simulink model "complete_plant"  (R2021b)
settings: Solver=VariableStepAuto  StartTime=0.0  StopTime=15  RelTol=1e-3
values from neighbouring files (symbols this model uses):
  a = Simulink.Parameter(1.14)    [startup.m]
  A1 = Simulink.Parameter(39.8344)    [startup.m]
  A2 = Simulink.Parameter(813.0780)    [startup.m]
  b = Simulink.Parameter(-0.03291)    [startup.m]
  B1 = Simulink.Parameter(0.000001287)    [startup.m]
  B2 = Simulink.Parameter(-0.002325)    [startup.m]
  B3 = Simulink.Parameter(3.797)    [startup.m]
  c = Simulink.Parameter(-1.14)    [startup.m]
  C1 = Simulink.Parameter(-0.000000002541)    [startup.m]
  C2 = Simulink.Parameter(0.000005279)    [startup.m]
  C3 = Simulink.Parameter(-0.003943)    [startup.m]
  C4 = Simulink.Parameter(3.634)    [startup.m]
  C_param = Simulink.Parameter([0 13757.41 21278.97 26666.02 30253.47 30313.18 30313.18])    [startup.m]
  d = Simulink.Parameter(-1.027)    [startup.m]
  driver_gain = 1    [startup.m]
  FZ_C = Simulink.Parameter([0 204.13 427.04 668.1 895.72 1124.40 1324.40])    [startup.m]
  gr = Simulink.Parameter([6.63043, 6.63043, 7.95652, 7.95652])    [startup.m]
  I = 15    [startup.m]
  inch2mm = Simulink.Parameter(25.4)    [startup.m]
  J_z = Simulink.Parameter(75)    [startup.m]
  k_limit = Simulink.Parameter(3.461)    [startup.m]
  Ku = Simulink.Parameter(0.24 / g.Value)    [startup.m]
  l = Simulink.Parameter([0.7922471, 0.7828529])    [startup.m]
  max_yaw_field = Simulink.Parameter([1.34 1.34 1.34 1.66 1.14 1.24 0.754 0.849 0.85 0.85])    [startup.m]
  min_speed_regen = Simulink.Parameter(85)    [startup.m]
  motor_efficiency = Simulink.Parameter([0.85, 0.85, 0.85, 0.85])    [startup.m]
  motor_limit_power = Simulink.Parameter([15000, 15000, 15000, 15000])    [startup.m]
  motor_limit_torque = Simulink.Parameter([-25, 25])    [startup.m]
  mu_factor = Simulink.Parameter(2/3)    [startup.m]
  P = 1    [startup.m]
  ramp_rate = 1    [startup.m]
  RE = Simulink.Parameter(0.2228169203)    [startup.m]
  s = Simulink.Parameter([0.647895, 0.62102])    [startup.m]
  S1 = Simulink.Parameter(7 * (10^(-5)))    [startup.m]
  S2 = Simulink.Parameter(-0.0038)    [startup.m]
  S3 = Simulink.Parameter(0.6535)    [startup.m]
  S4 = Simulink.Parameter(0.1061)    [startup.m]
  steer_slope = Simulink.Parameter(0.0111)    [startup.m]
  T = 0    [startup.m]
  T2F = Simulink.Parameter(single([29 29 35 35]))    [startup.m]
  tau = Simulink.Parameter(0)    [startup.m]
  time_delay = 0.022    [startup.m]
  V_target = Simulink.Parameter([0 3 6 9 12 15 18 21 25 31])    [startup.m]
undefined symbols (not defined in the file or in its folder): DiscIntNeverNeededParam
libraries: fl_lib x20, nesl_utility x12, sdl_lib x4, slpidlib x2, simulink x2, autolibdatasheetbattery x1, autolibmappedmotor x1, vehdynlibtire x1, autolibshared x1, vehdynlibviscommon x1
(part 3 of 4)

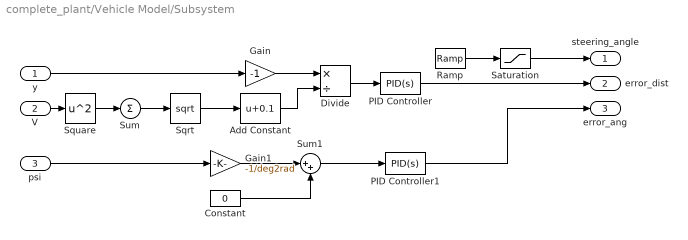
== system complete_plant/Vehicle Model/Subsystem ==
  y : Inport
  V : Inport  Port=2
  psi : Inport  Port=3
  Add Constant : Bias  Bias=0.1
  Constant : Constant  Value=0
  Divide : Product  Inputs=*/
  Gain : Gain  Gain=-1
  Gain1 : Gain  Gain=-1/deg2rad
  PID Controller : slpidlib/PID Controller  Controller=PID  Form=Parallel  TimeDomain=Continuous-time  UseExternalTs=off  SampleTime=-1  IntegratorMethod=Forward Euler  FilterMethod=Forward Euler  ControllerParametersSource=internal  P=50  I=0  D=2  UseFilter=on  N=50  TunerSelectOption=Transfer Function Based (PID Tuner App)  InitialConditionSource=internal  InitialConditionForIntegrator=0  InitialConditionForFilter=0  DifferentiatorICPrevScaledInput=0  ExternalReset=none  TrackingMode=off  Kt=1  LimitOutput=on  SatLimitsSource=internal  UpperSaturationLimit=40  LowerSaturationLimit=-40  LinearizeAsGain=on  AntiWindupMode=none  Kb=1  POutMin=[]  POutMax=[]  IOutMin=[]  IOutMax=[]  DOutMin=[]  DOutMax=[]  NOutMin=[]  NOutMax=[]  SumOutMin=[]  SumOutMax=[]  SaturationOutMin=[]  SaturationOutMax=[]  PParamMin=[]  PParamMax=[]  IParamMin=[]  IParamMax=[]  DParamMin=[]  DParamMax=[]  NParamMin=[]  NParamMax=[]  KbParamMin=[]  KbParamMax=[]  KtParamMin=[]  KtParamMax=[]  KbOutMin=[]  KbOutMax=[]  KtOutMin=[]  KtOutMax=[]  IntegratorOutMin=[]  IntegratorOutMax=[]  FilterOutMin=[]  FilterOutMax=[]  SumI1OutMin=[]  SumI1OutMax=[]  SumI2OutMin=[]  SumI2OutMax=[]  SumI3OutMin=[]  SumI3OutMax=[]  SumI4OutMin=[]  SumI4OutMax=[]  SumDOutMin=[]  SumDOutMax=[]  DifferentiatorOutMin=[]  DifferentiatorOutMax=[]  FilterDiffOutCoefMin=[]  FilterDiffOutCoefMax=[]  ReciprocalOutMin=[]  ReciprocalOutMax=[]  SumDenOutMin=[]  SumDenOutMax=[]  SumNumOutMin=[]  SumNumOutMax=[]  DivideOutMin=[]  DivideOutMax=[]  UdiffTsProdOutMin=[]  UdiffTsProdOutMax=[]  NTsProdOutMin=[]  NTsProdOutMax=[]  UintegralTsProdOutMin=[]  UintegralTsProdOutMax=[]  UngainTsProdOutMin=[]  UngainTsProdOutMax=[]  IntegratorContinuousStateAttributes=''  IntegratorStateMustResolveToSignalObject=off  IntegratorRTWStateStorageClass=Auto  FilterContinuousStateAttributes=''  FilterStateMustResolveToSignalObject=off  FilterRTWStateStorageClass=Auto  ParallelPVariant=InternalParameters  IdealPVariant=Disabled  IVariant=InternalParameters  DVariant=InternalParameters  IntegratorVariant=Continuous  SatVariant=Enabled  AWVariant=Passthrough  PCopyVariant=Disabled  TRVariant=Disabled  FdbkBlocksVariant=Forward  IdealPFdbkVariant=Disabled  SatFdbkVariant=Disabled  DerivativeFilterVariant=ContFilter  NVariant=InternalParameters  NCopyVariant=Disabled  FilterICVariant=InternalICsFilter  IntegratorICVariant=InternalICs  ExternalResetVariant=Disabled  TRSumVariant=Passthrough  SumFdbkVariant=Disabled  SumVariant=Sum_PID  TsampFilterVariant=InternalTs  TsampNgainVariant=Passthrough  TsampIntegralVariant=Passthrough  ExternalSaturationOutDataTypeStr=Inherit: Same as second input
  PID Controller1 : slpidlib/PID Controller  Controller=PID  Form=Parallel  TimeDomain=Continuous-time  UseExternalTs=off  SampleTime=-1  IntegratorMethod=Forward Euler  FilterMethod=Forward Euler  ControllerParametersSource=internal  P=0.4  I=0  D=0.8  UseFilter=on  N=35  TunerSelectOption=Transfer Function Based (PID Tuner App)  InitialConditionSource=internal  InitialConditionForIntegrator=0  InitialConditionForFilter=0  DifferentiatorICPrevScaledInput=0  ExternalReset=none  TrackingMode=off  Kt=1  LimitOutput=on  SatLimitsSource=internal  UpperSaturationLimit=40  LowerSaturationLimit=-40  LinearizeAsGain=on  AntiWindupMode=none  Kb=1  POutMin=[]  POutMax=[]  IOutMin=[]  IOutMax=[]  DOutMin=[]  DOutMax=[]  NOutMin=[]  NOutMax=[]  SumOutMin=[]  SumOutMax=[]  SaturationOutMin=[]  SaturationOutMax=[]  PParamMin=[]  PParamMax=[]  IParamMin=[]  IParamMax=[]  DParamMin=[]  DParamMax=[]  NParamMin=[]  NParamMax=[]  KbParamMin=[]  KbParamMax=[]  KtParamMin=[]  KtParamMax=[]  KbOutMin=[]  KbOutMax=[]  KtOutMin=[]  KtOutMax=[]  IntegratorOutMin=[]  IntegratorOutMax=[]  FilterOutMin=[]  FilterOutMax=[]  SumI1OutMin=[]  SumI1OutMax=[]  SumI2OutMin=[]  SumI2OutMax=[]  SumI3OutMin=[]  SumI3OutMax=[]  SumI4OutMin=[]  SumI4OutMax=[]  SumDOutMin=[]  SumDOutMax=[]  DifferentiatorOutMin=[]  DifferentiatorOutMax=[]  FilterDiffOutCoefMin=[]  FilterDiffOutCoefMax=[]  ReciprocalOutMin=[]  ReciprocalOutMax=[]  SumDenOutMin=[]  SumDenOutMax=[]  SumNumOutMin=[]  SumNumOutMax=[]  DivideOutMin=[]  DivideOutMax=[]  UdiffTsProdOutMin=[]  UdiffTsProdOutMax=[]  NTsProdOutMin=[]  NTsProdOutMax=[]  UintegralTsProdOutMin=[]  UintegralTsProdOutMax=[]  UngainTsProdOutMin=[]  UngainTsProdOutMax=[]  IntegratorContinuousStateAttributes=''  IntegratorStateMustResolveToSignalObject=off  IntegratorRTWStateStorageClass=Auto  FilterContinuousStateAttributes=''  FilterStateMustResolveToSignalObject=off  FilterRTWStateStorageClass=Auto  ParallelPVariant=InternalParameters  IdealPVariant=Disabled  IVariant=InternalParameters  DVariant=InternalParameters  IntegratorVariant=Continuous  SatVariant=Enabled  AWVariant=Passthrough  PCopyVariant=Disabled  TRVariant=Disabled  FdbkBlocksVariant=Forward  IdealPFdbkVariant=Disabled  SatFdbkVariant=Disabled  DerivativeFilterVariant=ContFilter  NVariant=InternalParameters  NCopyVariant=Disabled  FilterICVariant=InternalICsFilter  IntegratorICVariant=InternalICs  ExternalResetVariant=Disabled  TRSumVariant=Passthrough  SumFdbkVariant=Disabled  SumVariant=Sum_PID  TsampFilterVariant=InternalTs  TsampNgainVariant=Passthrough  TsampIntegralVariant=Passthrough  ExternalSaturationOutDataTypeStr=Inherit: Same as second input
  Ramp : simulink/Sources/Ramp  slope=10  start=2  InitialOutput=0
  Saturation : Saturate  UpperLimit=70
  Sqrt : Sqrt  SaturateOnIntegerOverflow=on
  Square : Math  Operator=square  SaturateOnIntegerOverflow=on
  Sum : Sum  Inputs=+
  Sum1 : Sum  Inputs=|++
  steering_angle : Outport
  error_dist : Outport  Port=2
  error_ang : Outport  Port=3
  wires:
  Add Constant/1 -> Divide/2
  V/1 -> Square/1
  Sum/1 -> Sqrt/1
  Sqrt/1 -> Add Constant/1
  Gain/1 -> Divide/1
  Constant/1 -> Sum1/2
  psi/1 -> Gain1/1
  Sum1/1 -> PID Controller1/1
  Divide/1 -> PID Controller/1
  Ramp/1 -> Saturation/1
  Square/1 -> Sum/1
  Gain1/1 -> Sum1/1
  y/1 -> Gain/1
  Saturation/1 -> steering_angle/1
  PID Controller/1 -> error_dist/1
  PID Controller1/1 -> error_ang/1

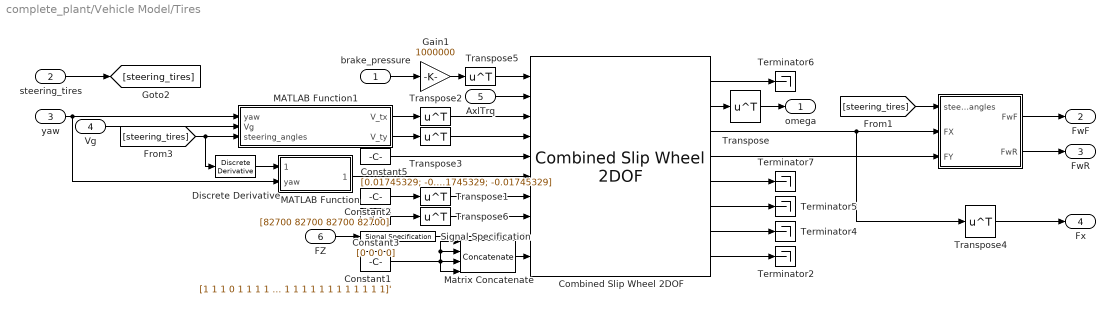
== system complete_plant/Vehicle Model/Tires ==
  brake_pressure : Inport
  steering_tires : Inport  Port=2
  yaw : Inport  Port=3
  Vg : Inport  Port=4
  AxlTrq : Inport  Port=5  PortDimensions=[4 1]
  FZ : Inport  Port=6
  " " : MATLAB Function  TreatAsAtomicUnit=on  SystemSampleTime=0.0005
  Combined Slip Wheel 2DOF : vehdynlibtire/Combined Slip Wheel 2DOF  tireType=Performance car 225/40R19  BrakeType=Disc  plySteer=off  turnslip=off  mu_static=.3  mu_kinetic=.2  disk_abore=.05  Rm=.177  num_pads=2  drum_abore=0.0508  drum_a=0.123  drum_c=0.212  drum_r=0.15  drum_theta1=0  drum_theta2=126  brake_p_bpt=[1 11.4736842105263 21.9473684210526 32.4210526315789 42.8947368421053 53.3684210526316 63.8421052631579 74.3157894736842 84.7894736842105 95.2631578947368 105.736842105263 116.210526315789 126.684210526316 137.157894736842 147.631578947368 158.105263157895 168.578947368421 179.052631578947 189.526315789474 200]  brake_n_bpt=[0 52.6315789473684 105.263157894737 157.894736842105 210.526315789474 263.157894736842 315.789473684211 368.421052631579 421.052631578947 473.684210526316 526.315789473684 578.947368421053 631.578947368421 684.210526315789 736.842105263158 789.473684210526 842.105263157895 894.736842105263 947.368421052632 1000]  f_brake_t=[43.4900602404453 42.5056030554862 41.5350898940194 40.5780454442085 39.6340111501808 38.7025443887544 37.7832176914519 36.8756180088306 35.9793460143796 35.0940154454303 34.2192524787115 33.3546951383474 32.4999927342521 31.6548053290159 30.8188032315107 29.991666515561 29.1730845621415 28.362755623661 27.5603864089927 26.765691687993;498.991217495636 487.695866636631 476.560505099801 465.579679307235 454.748127933653 444.060772460445 433.51270824929 423.099196101319 412.81565427025 402.657650900201 392.620896861006 382.701238955775 372.894653477208 363.197240090814 353.605216024701 344.114910546964 334.722759712992 325.425301366216 316.219170376863 307.10109410434;954.492374750826 932.886130217776 911.585920305583 890.581313170261 869.862244717126 849.419000532136 829.242198807128 809.322774193808 789.651962526121 770.221286354971 751.0225412433 732.047782773203 713.289314220164 694.739674852612 676.391628817892 658.238154578366 640.272434863842 622.48784710877 604.877954344734 587.436496520688;1409.99353200602 1378.07639379892 1346.61133551136 1315.58294703329 1284.9763615006 1254.77722860383 1224.97168936497 1195.5463522863 1166.48827078199 1137.78492180974 1109.42418562559 1081.39432659063 1053.68397496312 1026.28210961441 999.178041611083 972.361398609768 945.822110014692 919.550392851325 893.536738312604 867.771898937035;1865.49468926121 1823.26665738007 1781.63675071715 1740.58458089631 1700.09047828407 1660.13545667552 1620.7011799228 1581.76993037878 1543.32457903786 1505.34855726451 1467.82583000789 1430.74087040806 1394.07863570608 1357.82454437621 1321.96445440427 1286.48464264117 1251.37178516554 1216.61293859388 1182.19552228048 1148.10730135338;2320.9958465164 2268.45692096121 2216.66216592293 2165.58621475934 2115.20459506754 2065.49368474721 2016.43067048064 1967.99350847127 1920.16088729373 1872.91219271928 1826.22747439018 1780.08741422549 1734.47329644903 1689.36697913801 1644.75086719747 1600.60788667257 1556.92146031639 1513.67548433643 1470.85430624835 1428.44270376973;2776.49700377159 2713.64718454235 2651.68758112871 2590.58784862237 2530.31871185102 2470.8519128189 2412.16016103848 2354.21708656376 2296.9971955496 2240.47582817405 2184.62911877248 2129.43395804292 2074.86795719199 2020.9094138998 1967.53727999066 1914.73113070398 1862.47113546724 1810.73803007899 1759.51309021622 1708.77810618608;3231.99816102678 3158.8374481235 3086.71299633449 3015.58948248539 2945.43282863449 2876.21014089059 2807.88965159632 2740.44066465625 2673.83350380547 2608.03946362882 2543.03076315477 2478.78050186034 2415.26261793494 2352.4518486616 2290.32369278385 2228.85437473538 2168.02081061809 2107.80057582154 2048.17187418409 1989.11350860242;3687.49931828197 3604.02771170464 3521.73841154027 3440.59111634842 3360.54694541796 3281.56836896228 3203.61914215416 3126.66424274874 3050.66981206134 2975.60309908359 2901.43240753707 2828.12704567777 2755.6572786779 2683.9942834234 2613.11010557704 2542.97761876678 2473.57048576894 2404.8631215641 2336.83065815196 2269.44891101877;4143.00047553716 4049.21797528579 3956.76382674606 3865.59275021144 3775.66106220143 3686.92659703397 3599.34863271199 3512.88782084123 3427.50612031721 3343.16673453836 3259.83405191936 3177.4735894952 3096.05193942085 3015.5367181852 2935.89651837023 2857.10086279818 2779.12016091979 2701.92566730665 2625.48944211983 2549.78431343512;4598.50163279235 4494.40823886693 4391.78924195184 4290.59438407447 4190.77517898491 4092.28482510566 3995.07812326983 3899.11139893372 3804.34242857308 3710.73036999313 3618.23569630166 3526.82013331263 3436.44660016381 3347.079152947 3258.68293116342 3171.22410682959 3084.66983607064 2998.98821304921 2914.1482260877 2830.11971585147;5054.00279004754 4939.59850244808 4826.81465715762 4715.59601793749 4605.88929576838 4497.64305317735 4390.80761382767 4285.3349770262 4181.17873682896 4078.2940054479 3976.63734068395 3876.16667713006 3776.84126090677 3678.62158770879 3581.46934395661 3485.34735086099 ...(+2764 chars)]  tireParamSet=C:\Users\Inver\OneDrive\Desktop\TVS MATLAB\LCO_6in.tir  PRESMAX=1003118  PRESMIN=9982  FZMAX=10000  FZMIN=100  VXLOW=0.001  KPUMAX=1.5  KPUMIN=-1.5  ALPMAX=1.5708  ALPMIN=-1.5708  CAMMAX=0.173142086627737  CAMMIN=-0.173348165334087  LONGVL=16.7  FxRelFreqLwrLim=200*pi  FyRelFreqLwrLim=200*pi  MyRelFreqLwrLim=100*pi  omegao=0  br=1e-3  UNLOADED_RADIUS=0.2286  NOMPRES=83900  FNOMIN=1080  WIDTH=0.1524  RIM_RADIUS=.127  MASS=16.5  IYY=0.2966816056  GRAVITY=-9.81  zo=0  zdoto=0  BREFF=0.228  DREFF=0.222  FREFF=0.217  Q_RE0=0  Q_V1=0  Q_V2=0  Q_FZ1=0  Q_FZ2=0  Q_FZ3=0  Q_FCX=0  Q_FCY=0  Q_FCY2=0  PFZ1=0  VERTICAL_STIFFNESS=207885.061134007  VERTICAL_DAMPING=494.649255786991  BOTTOM_OFFST=.01  BOTTOM_STIFF=2e6  LONGITUDINAL_STIFFNESS=388714.175879854  LATERAL_STIFFNESS=157087.404633332  PCFX1=0  PCFX2=0  PCFX3=0  PCFY1=0  PCFY2=0  PCFY3=0  Q_RA1=0.675942571700787  Q_RA2=0.73800463546164  Q_RB1=1.04487486456705  Q_RB2=-1.191763806629  PCX1=1.5  PDX1=2.5435  PDX2=-0.64572  PDX3=10.9219  PEX1=-7.42e-13  PEX2=-0.70398  PEX3=0  PEX4=0  PKX1=42.5958  PKX2=0.0014247  PKX3=-0.55562  PHX1=0.0014842  PHX2=-0.0021096  PVX1=-0.075895  PVX2=0.1  PPX1=0.046916  PPX2=2.6527  PPX3=-0.025299  PPX4=-1.4293  RBX1=6.2196  RBX2=8.4467  RBX3=-138.4661  RCX1=0.89167  REX1=-4.5587  REX2=0.99676  RHX1=-0.057442  QSX1=0  QSX2=0  QSX3=0  QSX4=0  QSX5=0  QSX6=0  QSX7=0  QSX8=0  QSX9=0  QSX10=0  QSX11=0  QSX12=0  QSX13=0  QSX14=0  PPMX1=0  PCY1=1.5  PDY1=2.4332  PDY2=-0.5  PDY3=5.3003  PEY1=0.92478  PEY2=0.90262  PEY3=-3.7396e-07  PEY4=-0.00064548  PEY5=-0.034343  PKY1=-25.8914  PKY2=0.83173  PKY3=1  PKY4=2  PKY5=33.8601  PKY6=5.6535  PKY7=-0.37194  PHY1=-0.0026544  PHY2=-0.00020549  PVY1=-0.053073  PVY2=0.0054748  PVY3=1.242  PVY4=1.1283  PPY1=2  PPY2=-2  PPY3=-2  PPY4=0.8522  PPY5=0  RBY1=15.9574  RBY2=15.4039  RBY3=-0.047368  RBY4=-90  RCY1=1.0677  REY1=0.56886  REY2=-0.12642  RHY1=0.026731  RHY2=0.043261  RVY1=1.5319  RVY2=-11.6508  RVY3=-53.847  RVY4=-549.9496  RVY5=-0.0033543  RVY6=-13.8004  QSY1=0  QSY2=0  QSY3=0  QSY4=0  QSY5=0  QSY6=0  QSY7=0  QSY8=0  QBZ1=0  QBZ2=0  QBZ3=0  QBZ4=0  QBZ5=0  QBZ6=0  QBZ9=0  QBZ10=0  QCZ1=0  QDZ1=0  QDZ2=0  QDZ3=0  QDZ4=0  QDZ6=0  QDZ7=0  QDZ8=0  QDZ9=0  QDZ10=0  QDZ11=0  QEZ1=0  QEZ2=0  QEZ3=0  QEZ4=0  QEZ5=0  QHZ1=0  QHZ2=0  QHZ3=0  QHZ4=0  PPZ1=0  PPZ2=0  SSZ1=0  SSZ2=0  SSZ3=0  SSZ4=0  PDXP1=0  PDXP2=0  PDXP3=0  PKYP1=0  PDYP1=0  PDYP2=0  PDYP3=0  PDYP4=0  PHYP1=0  PHYP2=0  PHYP3=0  PHYP4=0  PECP1=0  PECP2=0  QDTP1=0  QCRP1=0  QCRP2=0  QBRP1=0  QDRP1=0  QDRP2=0  aMode=2
      settings: SourceProductBaseCode=VE
  Constant1 : Constant  Value=[1 1 1 0 1 1 1 1 1 1 1 1 1 1 1 1 1 1 1 1 1 1 1 1 1 1 1]'  VectorParams1D=off
  Constant2 : Constant  Value=[82700 82700 82700 82700]  VectorParams1D=off
  Constant3 : Constant  Value=[0 0 0 0]  VectorParams1D=off
  Constant5 : Constant  Value=[0.01745329; -0.01745329; 0.01745329; -0.01745329]  VectorParams1D=off
  Discrete Derivative : simulink/Discrete/Discrete Derivative  gainval=1  ICPrevScaledInput=0.0  OutMin=[]  OutMax=[]  OutDataType=fixdt(1, 16)  OutScaling=2^-10  DoSatur=off
  Gain1 : Gain  Gain=1000000
  MATLAB Function : MATLAB Function  TreatAsAtomicUnit=on  SystemSampleTime=0.0005
  MATLAB Function1 : MATLAB Function  TreatAsAtomicUnit=on  SystemSampleTime=0.0005
  Matrix Concatenate : Concatenate  NumInputs=4  Mode=Multidimensional array  ConcatenateDimension=2
  Signal Specification : SignalSpecification  Dimensions=[4 1]
  Terminator{2,4..7} (5 alike) : Terminator
  Transpose{,1..6} (7 alike) : Math  Operator=transpose  SaturateOnIntegerOverflow=on
  omega : Outport
  FwF : Outport  Port=2
  FwR : Outport  Port=3
  Fx : Outport  Port=4
  wires:
  Combined Slip Wheel 2DOF/1 -> Terminator6/1
  Transpose1/1 -> Combined Slip Wheel 2DOF/7
  Constant5/1 -> Combined Slip Wheel 2DOF/5
  Constant1/1 -> Matrix Concatenate/4, Matrix Concatenate/1, Matrix Concatenate/2, Matrix Concatenate/3
  " "/1(FwF) -> FwF/1
  Matrix Concatenate/1 -> Combined Slip Wheel 2DOF/10
  FZ/1 -> Signal Specification/1
  Constant2/1 -> Transpose1/1
  Combined Slip Wheel 2DOF/5 -> Terminator7/1
  Combined Slip Wheel 2DOF/6 -> Terminator5/1
  Signal Specification/1 -> Combined Slip Wheel 2DOF/9
  Vg/1 -> MATLAB Function1/2(Vg)
  MATLAB Function/1(tire_yaw) -> Combined Slip Wheel 2DOF/6
  Combined Slip Wheel 2DOF/8 -> Terminator2/1
  Combined Slip Wheel 2DOF/7 -> Terminator4/1
  " "/2(FwR) -> FwR/1
  Transpose6/1 -> Combined Slip Wheel 2DOF/8
  Combined Slip Wheel 2DOF/4 -> " "/3(FY)
  MATLAB Function1/2(V_ty) -> Transpose3/1
  MATLAB Function1/1(V_tx) -> Transpose2/1
  AxlTrq/1 -> Combined Slip Wheel 2DOF/2
  Constant3/1 -> Transpose6/1
  Transpose3/1 -> Combined Slip Wheel 2DOF/4
  Combined Slip Wheel 2DOF/3 -> Transpose4/1, " "/2(FX)
  Transpose2/1 -> Combined Slip Wheel 2DOF/3
  yaw/1 -> MATLAB Function/2(yaw), MATLAB Function1/1(yaw)
  steering_tires/1 -> [steering_tires]
  [steering_tires] -> Discrete Derivative/1, MATLAB Function1/3(steering_angles)
  [steering_tires] -> " "/1(steering_angles)
  Combined Slip Wheel 2DOF/2 -> Transpose/1
  Transpose/1 -> omega/1
  Transpose5/1 -> Combined Slip Wheel 2DOF/1
  Gain1/1 -> Transpose5/1
  brake_pressure/1 -> Gain1/1
  Discrete Derivative/1 -> MATLAB Function/1(steer_yaw)
  Transpose4/1 -> Fx/1

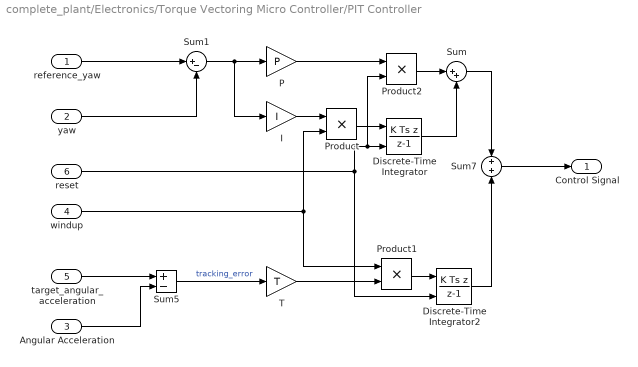
== system complete_plant/Electronics/Torque Vectoring Micro Controller/PIT Controller ==
  reference_yaw : Inport
  yaw : Inport  Port=2
  Angular Acceleration : Inport  Port=3
  windup : Inport  Port=4
  target_angular_acceleration : Inport  Port=5
  reset : Inport  Port=6
  Discrete-Time Integrator : DiscreteIntegrator  IntegratorMethod=Integration: Backward Euler  gainval=1  ExternalReset=falling  SampleTime=-1  ICPrevOutput=DiscIntNeverNeededParam  ICPrevScaledInput=DiscIntNeverNeededParam
  Discrete-Time Integrator2 : DiscreteIntegrator  IntegratorMethod=Integration: Backward Euler  gainval=1  ExternalReset=falling  SampleTime=-1  ICPrevOutput=DiscIntNeverNeededParam  ICPrevScaledInput=DiscIntNeverNeededParam
  I : Gain  Gain=I
  P : Gain  Gain=P
  Product : Product
  Product1 : Product
  Product2 : Product
  Sum : Sum  Inputs=|++
  Sum1 : Sum  Inputs=|+-
  Sum5 : Sum  Inputs=+-
  Sum7 : Sum
  T : Gain  Gain=T
  Control Signal : Outport
  wires:
  Sum5/1 -> T/1  "tracking_error"
  Sum/1 -> Sum7/1
  windup/1 -> Product1/1, Product/2
  Product/1 -> Discrete-Time Integrator/1
  I/1 -> Product/1
  Discrete-Time Integrator2/1 -> Sum7/2
  reference_yaw/1 -> Sum1/1
  yaw/1 -> Sum1/2
  Sum1/1 -> I/1, P/1
  Discrete-Time Integrator/1 -> Sum/2
  target_angular_acceleration/1 -> Sum5/1
  Angular Acceleration/1 -> Sum5/2
  T/1 -> Product1/2
  Product1/1 -> Discrete-Time Integrator2/1
  reset/1 -> Product2/2, Discrete-Time Integrator/2, Discrete-Time Integrator2/2
  P/1 -> Product2/1
  Product2/1 -> Sum/1
  Sum7/1 -> Control Signal/1

== matlab function complete_plant/Vehicle Model/Motor and Battery/Conditioner ==
  data: Tx input; Tx output
function Tx = conditioner(Tx)

if (Tx(1) - Tx(2)) < 0.2
    min_FTx = min(Tx(1:2));
    Tx(1) = min_FTx;
    Tx(2) = min_FTx;
end

if (Tx(3) - Tx(4)) < 0.2
    min_RTx = min(Tx(3:4));
    Tx(3) = min_RTx;
    Tx(4) = min_RTx;
end

end

== matlab function complete_plant/Electronics/Torque Vectoring Micro Controller/Constraint Generation ==
  data: power_limit output; lb output size=[1 4]; ub output size=[1 4]; A output size=[1 4]; b output size=1; Aeq output size=[1 4]; beq output size=1; y output size=[1 4]; target_ang_accel output size=1; windup output size=1; previous_Tx input size=[1 4]; driver_input input; power_limits_battery input; omega input size=[1 4]; steering input; Fx_max input; FY input; T_brake input; control_signal input; prev_plb input; motor_limit_power parameter; motor_efficiency parameter; J_z parameter; gr parameter; RE parameter; tau parameter; motor_limit_torque parameter; t parameter; l parameter; s parameter; T2F parameter; min_speed_regen parameter; power_limit_battery output; integrator_reset output; omega_m output size=[1 4]
function [power_limit, lb, ub, A, b, Aeq, beq, y, target_ang_accel, windup, power_limit_battery, integrator_reset, omega_m] = constraint_generation(previous_Tx, driver_input, power_limits_battery, omega, steering, Fx_max, FY, T_brake, control_signal, prev_plb,motor_limit_power, motor_efficiency, J_z, gr, RE, tau, motor_limit_torque, t, l, s, T2F, min_speed_regen)
%% Layer 2 Computation
% Developer(s):    David Farell
%                  Demetrius Gulewicz
%                  Elliot Stockwell
%                  Tao Sun
%
% Developed for: Purdue Electric Racing
% Date:          12/25/2021
%
% Description: This function primarily computes the maximum and minimum
%              torque that can be requested, based on slip, power, and 
%              transient constraints. Also computes yaw error.
%
%
%% Pass Through Signals
% prev_torque - Torque requested to motor in previous time step [Nm][4x1]
% driver_input - Proportion Of Total Available Power To Use [Unitless][1x1]
% FY - Tires Forces y Direction, Tire Fixed Coordinates [N][4x1]
%
%
%% Input Only
% power_limits_battery - Max & Min Total Battery Power Output [W][2x1]
% center_steer_angle - Steering Column Angle From Neutral [rad][1x1]
% acker_steer_angles - Angle Tires Are Turned From Neutral [rad][2x1]
% Fx_max - Max Tire Forces x Direction, Tire Fixed Coordinates [N][1x4]
% omega_w - Angular Velocity Of Tires, Tire Fixed Coordinates [m/s][1x4]
% yaw - Yaw Rate z Direction, Vehicle Fixed Coordinates  [rad/s][1x1]
% T_brake - Mechanical Brake Torque On Each Tire [Nm][1x4]
% yaw_ref - The Desired & Max Allowed Yaw Rate [rad/s][1x2]
%
%
%% Output Only
% power_limit_battery - Max OR Min Total Battery Power Output [W][1x1]
% omega_m - Motor Shaft Angular Velocity [rad/s][1x4]
% x - Equivalent Distances That Fx Acts From CoG [m][1x4]
% y - Equivalent Distances That Fy Acts From CoG [m][1x4] 
% slip_limit - Max Torque Before Tire Slips [Nm][1x4]
% torque_limit_motor - Max Torque Motor Can Output [Nm][1x4]
% tau_limit_upper - Max Torque Motor Is Allowed To Change To [Nm][1x4]
% tau_limit_lower - Min Torque Motor Is Allowed To Change To [Nm][1x4]
% yaw_err - Error Between Target & Actual Yaw Rate [rad/s][1x1]
% RPM_limit - Max Torque Possible at Current RPM [Nm][1x4]
%
%
%% Constants
% global s; % Half track width [m][1x2]
% global l; % Wheelbase [m][1x2]
% global motor_limit_power; % Absolute Power Limit For Each Motor [W][1x4]
% global motor_efficiency; % Motor Efficiency [Unitless][1x4]
% global tau; % Motor Response Time Constant [s][1x1]
% global t; % Controller Timing [s][1x1]
% global gr; % Gear Ratios [Unitless][1x4]
% global r; % Tire Radius [m][1x1]
% T2F - Convert Torque At The Motor Shaft to Force At The Tire [1/m][1x4]
% global motor_limit_torque; % Min & Max Torque Request From Motor [Nm][1x2]


%% Moment Arm For Tire Forces
% Calculate K_1 Vehicle Constants
x_1 = (s(1) * cos(steering(2))) + (l(1) * sin(steering(2)));
x_2 = (-1 * s(1) * cos(steering(3))) + (l(1) * sin(steering(3)));
x_3 = s(2);
x_4 = -s(2);
x = [x_1, x_2, x_3, x_4]; 

% Calculate K_2 Vehicle Constants
y_1 = (-1 * s(1) * sin(steering(2))) + (l(1) * cos(steering(2)));    
y_2 = (s(1) * sin(steering(3))) + (l(1) * cos(steering(3)));
y_3 = -l(2);
y_4 = -l(2);
y = [y_1, y_2, y_3, y_4]; 


%% Slip Limit
% Calculate Torque Limit Due to Power and Slip
slip_limit = (Fx_max-(T_brake./RE)) ./ T2F; 


%% Power Limit
% Motor Shaft Speed, RAD/S
omega_m = omega .* gr;

% % If torque_limit_motor ever exceed 30, then the exact value is no longer
% needed. As in, the ceiling is 30
power_limit = (motor_limit_power .* motor_efficiency) ./ omega_m;

% Erase power limit solution above torque limit, for better data
% visualization
for i = 1:4
    if power_limit(i) > 25 
        power_limit(i) = 25;
    elseif power_limit(i) < -25 && omega_m(i) > min_speed_regen
        power_limit(i) = -25; 
    elseif power_limit(i) < -25 && omega_m(i) > 0
        power_limit(i) = -0.01; 
    elseif power_limit(i) < -25 && omega_m(i) < 0
        power_limit(i) = 25; 
    end
end


%% RPM Limit
% This section in practice will probably just be a lookup table, when PER
% gets the chance to get test results for the motors
% Motor Shaft Speed, rpm
ang_vel_RPM = omega_m .* 9.5492965964254;

% quadratic constants that connect current and max RPM of motors
a_v = 0.2667;
b_v = -66.353;
c_v = 10452 - ang_vel_RPM;

% quadratic constants that connnect current and max torque of motors
a_t = -0.0987;
b_t = 45.799;
c_t = -129.65;

% maximum possible current at the current RPM
max_current = [0, 0, 0, 0];

% calculate the maximum current possible at the current RPM
for i = [1:4]
   if ang_vel_RPM(i) < 7000
       max_current(i) = 70;
   else
       max_current(i) = (-b_v - sqrt(b_v^2 - (4*a_v.*c_v(i)))) .* (1/(2*a_v));
   end
end

% calculate the maximum torque at the max current
rpm_limit = ((a_t .* (max_current.^2)) + (b_t .* max_current) + c_t) ./ 100;
for i = [1:4]
   if rpm_limit(i) < 0
      rpm_limit(i) = 0;
   end
end


%% Motor Response Limit
% Calculate Constants for getting limit on motor output torque due to
% motor response time
% Note: This section is only for simulation
e_term = exp(-t / tau);
c_lower = (1 - e_term) .* motor_limit_torque(1);
c_upper = (1 - e_term) .* motor_limit_torque(2);
c_constant = (previous_Tx .* e_term);

% Max and Min Torque Limits due to motor response time
tau_limit_upper = max([c_upper + c_constant; c_constant + .01]);
tau_limit_lower = min([c_lower + c_constant; c_constant - .01]);


%% Overall Power Limit
% If driver is not pressing acceleration pedal, no positive torque is allowed
if driver_input <= 0
   power_limit_battery = power_limits_battery(2);
else
    power_limit_battery = power_limits_battery(1);
end


%% Optimization Setup
% Calculate Boundary Conditions, The Max and Min Allowable Torque
ub = single([0, 0, 0, 0]);
lb = single([0, 0, 0, 0]);

for i = 1:4
    ub(i) = min([slip_limit(i), power_limit(i), motor_limit_torque(2), tau_limit_upper(i), rpm_limit(i)]);
    lb(i) = max([-slip_limit(i), -power_limit(i), motor_limit_torque(1), tau_limit_lower(i)]);
end

% Enforce No Backwards Rotation Of Tires
for i = 1:4
   if omega_m(i) < min_speed_regen && lb(i) < 0
       lb(i) = 0.001;
   end
end

% Max & Min Forces on the Tires
ub_f = ub .* T2F;
lb_f = lb .* T2F;

% Find Max & Min For PID, The Yaw Acceleration Of The Car
M_max=zeros(1,2);
M_max(1) = (x(1)*ub_f(1)+x(3)*ub_f(3)+x(2)*lb_f(2)+x(4)*lb_f(4)+sum(y.*FY))/J_z;
M_max(2) = (x(2)*ub_f(2)+x(4)*ub_f(4)+x(1)*lb_f(1)+x(3)*lb_f(3)+sum(y.*FY))/J_z;

% Limit PID To Be No Larger Than Possible Due To Torque Constraints
if control_signal >= M_max(1)
    control_signal = M_max(1);
    windup = 0;
elseif control_signal <= M_max(2)
    control_signal = M_max(2);
    windup = 0;
else
    windup = 1;
end

if control_signal >= 40
    control_signal = 40;
    windup = 0;
elseif control_signal <= -40
    control_signal = -40;
    windup = 0;
end

% Calculate Yaw Constraint
Aeq = ((1 ./ J_z) .* x) .* T2F;
beq = single(control_signal-sum(((1 / J_z) * y) .* FY));

if abs(beq) < 0.0001
    beq = single(0.0000001);
end

A = single(omega_m ./ motor_efficiency);
b = single(driver_input*power_limit_battery);

if (omega(4) < min_speed_regen) && (driver_input <= 0)
    control_signal = 0;
end

if sign(prev_plb) ~= sign(power_limit_battery)
    integrator_reset = 0;
else
    integrator_reset = 1;
end


target_ang_accel = control_signal;

end

== matlab function complete_plant/Vehicle Model/   ==
  data: Vg input; Fext output
function Fext = get_downforce(Vg)
%% Constants
rho = 1.225; % Air density [Kg/m^3]
cl = 2.11014; % Lift coefficient [unitless]
A = 1.0221; % Frontal Area [m^2]


%% Computation
% Compute CoG Velocity
Vcog = norm(Vg);

% Compute DownForce
Fz = 0.5 * rho * Vcog * cl * A;
Fext = [0, 0, Fz];

== matlab function complete_plant/Vehicle Model/Tires/MATLAB Function ==
  data: steer_yaw input; tire_yaw output; yaw input
function tire_yaw = fcn(steer_yaw, yaw)
tire_yaw = -[steer_yaw(1); steer_yaw(2); 0; 0] - yaw;
end

== matlab function complete_plant/Vehicle Model/Tires/  ==
  data: steering_angles input; FX input; FY input; FwF output size=[2 2]; FwR output size=[2 2]
function [FwF, FwR] = fcn(steering_angles, FX, FY)
%% Force Transformation, Tire Coordinates to Vehicle Coordinates
FX_FL  = (FX(1) .* cos(steering_angles(1))) + (FY(1) .* sin(steering_angles(1)));
FX_FR  = (FX(2) .* cos(steering_angles(2))) + (FY(2) .* sin(steering_angles(2)));

FY_FL = (FX(1) .* sin(steering_angles(1))) - (FY(1) .* cos(steering_angles(1)));
FY_FR = (FX(2) .* sin(steering_angles(2))) - (FY(2) .* cos(steering_angles(2)));


%% Construct Force Matrix
FwF = [[FX_FL; FY_FL] [FX_FR; FY_FR]];
FwR = [FX(3:4)'; -FY(3:4)'];

input = [FY'; FX'];

transform_matrix_FL = [cos(steering_angles(1)) sin(steering_angles(1)); -sin(steering_angles(1)) cos(steering_angles(1))];
transform_matrix_FR = [cos(steering_angles(2)) sin(steering_angles(2)); -sin(steering_angles(2)) cos(steering_angles(2))];
transform_matrix_RL = [cos(0) sin(0); -sin(0) cos(0)];
transform_matrix_RR = [cos(0) sin(0); -sin(0) cos(0)];

FX_FL = transform_matrix_FL * input(:, 1);
FX_FR = transform_matrix_FR * input(:, 2);
FX_RL = transform_matrix_RL * input(:, 3);
FX_RR = transform_matrix_RR * input(:, 4);

FwF = [FX_FL(2) -FX_FL(1); FX_FR(2) -FX_FR(1)];
FwR = [FX_RL(2) -FX_RL(1); FX_RR(2) -FX_RR(1)];

== matlab function complete_plant/Vehicle Model/Compute Anti-Ackermann ==
  data: steering_angle input; error_dist input; error_ang input; steering_tires output size=[1 2]; S1 parameter; S2 parameter; S3 parameter; S4 parameter; inch2mm parameter; steer_slope parameter; deg2rad parameter; error output
function [steering_tires, error]  = anti_ackermann(steering_angle, error_dist,  error_ang,S1, S2, S3, S4, inch2mm, steer_slope, deg2rad)
%% Inputs
% steering_angle                  [deg]


%% Outputs
% all_steering_angles             [rad][1x3]
%     steering_angle                  
%     left_steering_angle             
%     right_steering_angle            

%% Compute
if abs(error_dist) > abs(error_ang)
    error = (sign(error_dist)*(abs(error_dist) - abs(error_ang)))+error_ang;
else
    error = error_ang;
end

rack_displacement = steer_slope * inch2mm * error;

left_steering_angle = -((S1*(-rack_displacement)^3)+(S2*(-rack_displacement)^2)+(S3*-rack_displacement)+S4)*deg2rad;
right_steering_angle = ((S1*(rack_displacement)^3)+(S2*(rack_displacement)^2)+(S3*rack_displacement)+S4)*deg2rad;

steering_tires = [left_steering_angle, right_steering_angle];
end

== matlab function complete_plant/Electronics/Torque Vectoring Micro Controller/Normal Force Model ==
  data: temp_FZ input size=[1 4]; FZ output size=[1 4]; shock_displacement input size=[1 4]; shock_velocity input size=[1 4]
function FZ = normal_force_model(temp_FZ, shock_displacement, shock_velocity)
%% Inputs
% temp_FZ                  [N]
% shock_displacement       [m]
% shock_velocity           [m/s]


%% Outputs
% FZ                       [N]


%% Compute
FZ = temp_FZ;
end

== matlab function complete_plant/Electronics/Torque Vectoring Micro Controller/Steering Model ==
  data: steering_angle input size=1; steering output size=[1 3]; steer_slope parameter size=1; inch2mm parameter size=1; deg2rad parameter size=1; S1 parameter size=1; S2 parameter size=1; S3 parameter size=1; S4 parameter size=1
function steering  = steering_model(steering_angle, steer_slope, inch2mm, deg2rad, S1, S2, S3, S4)
%% Inputs
% steering_angle                  [deg]


%% Outputs
% all_steering_angles             [rad][1x3]
%     steering_angle                  
%     left_steering_angle             
%     right_steering_angle            

%% Compute
rack_displacement = steer_slope * inch2mm * steering_angle;

left_steering_angle = -((S1*(-rack_displacement)^3)+(S2*(-rack_displacement)^2)+(S3*-rack_displacement)+S4)*deg2rad;
right_steering_angle = ((S1*(rack_displacement)^3)+(S2*(rack_displacement)^2)+(S3*rack_displacement)+S4)*deg2rad;
steering_angle = (left_steering_angle + right_steering_angle) / 2;

steering = [steering_angle, left_steering_angle, right_steering_angle];
end

== matlab function complete_plant/Electronics/Torque Vectoring Micro Controller/Reference Generation ==
  data: reference_yaw output size=1; steering_angles input size=1; V input size=[1 2]; l parameter size=[1 2]; Ku parameter size=1; V_target parameter size=[1 10]; max_yaw_field parameter size=[1 10]
function reference_yaw = reference_generation(steering_angles, V, l, Ku, V_target, max_yaw_field)
%% Inputs
% all_steering_angles      [rad][1x3]
%     steering_angle                  
%     left_steering_angle             
%     right_steering_angle   
% Vg                       [m/s][1x2]
%    Vx
%    Vy


%% Outputs
% reference_yaw            [N]


%% Compute
% Yaw Calculations
% If yaw_des or yaw_max ever exceed 3, then the exact value is no longer
% needed. As in, the ceiling of these two variables is 3.

v_cog = norm(V);
yaw_max = pchip(V_target, max_yaw_field,v_cog);
yaw_des = (v_cog * steering_angles) / ((l(1) + l(2)) + (Ku * v_cog ^ 2));

% Modified
yaw_ref_potentials = [yaw_des, yaw_max];

% Calculate the Yaw Error, Apply Sign Convention
if yaw_des == 0
    reference_yaw = 0;
else
    reference_yaw = sign(yaw_des) * min(abs(yaw_ref_potentials));
end
end

== matlab function complete_plant/Electronics/Torque Vectoring FPGA/Optimization  ==
  settings: updateMethod=DISCRETE
  data: previous_Tx input size=[1 4]; Tx_actual output double size=[1 4]; driver_input input size=1; omega input size=[1 4]; min_speed_regen parameter size=1; bigM_flag output size=1; typed output size=1; lb input size=[1 4]; ub input size=[1 4]; A input size=[1 4]; b input size=1; Aeq input size=[1 4]; beq input size=1; T2F parameter size=[1 4]; gr parameter size=[1 4]
function [Tx_actual, bigM_flag, typed] = optimization(previous_Tx, driver_input, omega, min_speed_regen, lb, ub, A, b, Aeq, beq, T2F, gr)
%% LP_calc Computation
% Developer(s):    David Farell
%                  Demetrius Gulewicz
%                  Elliot Stockwell
%                  Tao Sun
%
% Developed for: Purdue Electric Racing
% Date:          12/25/2021
%
% Description: This function primarily computes the desired torque
%              distribution after constructing an optimization statement.
%
%
%% Pass Through Signals
% omega_m - Motor Shaft Angular Velocity [rad/s][1x4]
%
%
%% Input Only
% prev_torque - Torque Requested To Motor In Previous Time Step [Nm][4x1]
% driver_input - Proportion of total available power to use [Unitless][1x1]
% T2F - Convert Torque At The Motor Shaft to Force At The Tire [1/m][1x4]
% power_limit_battery - Max & Min Total Battery Power Output [W][1x2]
% FY - Tires Forces y Direction, Tire fixed coordinates [N][1x4]
% x - Equivalent Distances That FX Acts From CoG [m][1x4]
% y - Equivalent Distances That FY Acts From CoG [m][1x4]
% slip_limit - Max Torque Before Tire Slips [Nm][1x4]
% torque_limit_motor - Max Torque Motor Can Output [Nm][1x4]
% tau_limit_upper - Max Torque Motor Is Allowed To Change To [Nm][1x4]
% tau_limit_lower - Min Torque Motor Is Allowed To Change To [Nm][1x4]
% PID - Desired Yaw Acceleration [rad/s^2][1x1]
%
%
%% Output Only
% Tx - Torque Request To Motors [Nm][4x1]
% lb - Min Torque Request [Nm][1x4]
% ub - Max Torque Request [Nm][1x4]
% Aeq - Moment About CoG, Optimization Variable [rad/s^2][1x1]
% beq - Moment About CoG, Yaw Acceleration & Other Foces [rad/s^2][1x1]
% A - Power Consumed, Optimization Variable [W][1x1]
% b - Power Consumed, Driver Input [W][1x1]
% M_max - Max & Min Yaw Acceleration Achievable With lb & ub [rad/s^2][1x2]
% Power - Total Estimated Power Consumed by the 4 Motors
% TR - The Estimated Yaw Acceleration from the Vehicle
%
%
%% Constants
% global J_z; % Polar Moment Of Inertia [kg m^2][1x1]
% global motor_efficiency; % Motor efficiency [Unitless][1x4]
% global motor_limit_torque; % Minimum & Max Torque Request From Motor [Nm][1x2]
% global min_speed_regen; % Min Motor Shaft Speed For Regen Braking [rad/s][1x1]
% T2F - Convert Torque At The Motor Shaft to Force At The Tire [1/m][1x4]


%% Temporary
min_omegas = min(omega.*gr);
min_omega = min_omegas(1);


%% Detect Potential Zero Crossing, Determine Augmented lb and ub
lb_plus = lb;
ub_neg = ub;
zero_crossing = 0;
crossing_locations = [0 0 0 0];
yaw_error_limit = 0.2;

for i = 1:4
    if lb_plus(i) < 0 && ub_neg(i) > 0
        zero_crossing = 1;
        crossing_locations(i) = i;
        
        if sign(previous_Tx(i)) > 0
            lb_plus(i) = 0.001;
        elseif sign(previous_Tx(i)) < 0
            ub_neg(i) = -0.001;          
        end
    elseif abs(ub(i) - lb(i)) < 0.5
        ub_neg(i) = -0.001; 
        lb_plus(i) = -10;
        lb(i) = -0.002;
        ub(i) = 0.002;
    end
end

signs = sign(lb_plus);
             
%% Optimization
Tx = single([0 0 0 0]);
bigM_flag = single(0);
typed = 0;
ub_adjust = [0 0 0 0];
lb_adjust = [0 0 0 0];

signs_adjust = [0 0 0 0];

if driver_input < 0
    T2F_aug = -T2F;
    A = -A;
else
    T2F_aug = T2F;
end

if ~(min_omega < min_speed_regen && driver_input < 0)
    if (zero_crossing == 1 && min_omega > 10)
            % Zero Crossing Primary Optimization
            [Tx21, Tx22, Tx23, Tx24, bigM_flag2] = call_bigM_C(T2F_aug, b, A, beq, Aeq, lb_plus, ub_neg, signs, yaw_error_limit);           
            Tx2 = double([Tx21, Tx22, Tx23, Tx24]);
            
            for i = 1:4
                if abs(Tx2(i)) < 0.002 && abs(Tx2(i)) >= 0.001 && crossing_locations(i) > 0
                    if signs(i) > 0
                        lb_adjust(i) = lb(i);
                        ub_adjust(i) = -lb_plus(i);
                    else
                        lb_adjust(i) = -ub_neg(i);
                        ub_adjust(i) = ub(i);  
                    end
                elseif crossing_locations(i) > 0
                    lb_adjust(i) = lb_plus(i);
                    ub_adjust(i) = ub_neg(i);
                else
                    lb_adjust(i) = lb(i);
                    ub_adjust(i) = ub(i);
                end
            end
            
            signs_adjust = sign(lb_adjust);
            [Tx31, Tx32, Tx33, Tx34, bigM_flag3] = call_bigM_C(T2F_aug, b, A, beq, Aeq, lb_adjust, ub_adjust, signs_adjust, yaw_error_limit);
            Tx3 = double([Tx31, Tx32, Tx33, Tx34]);
            
            % Zero Crossing Secondary Optimization
%             [Tx5, bigM_flag5] = call_bigM_alt(b, A, beq, Aeq, lb, ub_neg);
%             
%             for i = 1:4
%                 if abs(Tx5(i)) < 0.002 && abs(Tx5(i)) >= 0.001 && crossing_locations(i) > 0
%                     if signs(i) > 0
%                         lb_adjust(i) = lb(i);
%                         ub_adjust(i) = -lb_plus(i);
%                     else
%                         lb_adjust(i) = -ub_neg(i);
%                         ub_adjust(i) = ub(i);  
%                     end
%                 elseif crossing_locations(i) > 0
%                     lb_adjust(i) = lb_plus(i);
%                     ub_adjust(i) = ub_neg(i);
%                 else
%                     lb_adjust(i) = lb(i);
%                     ub_adjust(i) = ub(i);
%                 end
%             end
%             
%             [Tx6, bigM_flag6] = call_bigM_alt(b, A, beq, Aeq, lb_adjust, ub_adjust);
            
            % Optimization Selection
            if bigM_flag3 == 1 || bigM_flag3 == 3
                Tx = single(Tx3);
                typed = 3;
                bigM_flag = single(bigM_flag3);
            else
                Tx = single(previous_Tx);
                typed = 6;
                bigM_flag = single(bigM_flag3);
            end
    else    
        % No Zero Crossing
        [Tx11, Tx12, Tx13, Tx14, bigM_flag1] = call_bigM_C(T2F_aug, b, A, beq, Aeq, lb, ub, signs, 0.05);
        Tx1 = [Tx11, Tx12, Tx13, Tx14];
%         [Tx4, bigM_flag4] = call_bigM_alt(b, A, beq, Aeq, lb, ub);
        
        % Optimization Selection
        if bigM_flag1 == 3 || bigM_flag1 == 1
            Tx = single(Tx1);
            typed = 1;
            bigM_flag = single(bigM_flag1);
        else
            Tx = single(previous_Tx);
            typed = 4;
            bigM_flag = single(bigM_flag1);
        end   
    end
else
    typed = 7;
    bigM_flag = single(3);
end

Tx_actual = double(Tx);


%% Simplified Control Scheme
% Tx_actual = driver_input .* [25; 25; 25; 25];


end

== matlab function complete_plant/Vehicle Model/Tires/MATLAB Function1 ==
  data: yaw input; V_tx output size=[1 4]; Vg input; steering_angles input; s parameter; l parameter; V_ty output size=[1 4]
function [V_tx, V_ty] = get_tire_velocities(yaw, Vg, steering_angles, s, l)
V_fl = Vg + (yaw .* [s(1) l(1)]);
V_fr = Vg + (yaw .* [-s(1) l(1)]);
V_rl = Vg + (yaw .* [s(2) -l(2)]);
V_rr = Vg + (yaw .* [-s(2) -l(2)]);

V_x = [V_fl(1) V_fr(1) V_rl(1) V_rr(1)];
V_y = [V_fl(2) V_fr(2) V_rl(2) V_rr(2)];

steering_angles = -steering_angles;

input = [V_y; V_x];

transform_matrix_FL = [cos(steering_angles(1)) sin(steering_angles(1)); -sin(steering_angles(1)) cos(steering_angles(1))];
transform_matrix_FR = [cos(steering_angles(2)) sin(steering_angles(2)); -sin(steering_angles(2)) cos(steering_angles(2))];
transform_matrix_RL = [cos(0) sin(0); -sin(0) cos(0)];
transform_matrix_RR = [cos(0) sin(0); -sin(0) cos(0)];

V_FL = transform_matrix_FL * input(:, 1);
V_FR = transform_matrix_FR * input(:, 2);
V_RL = transform_matrix_RL * input(:, 3);
V_RR = transform_matrix_RR * input(:, 4);

V_tx = [V_FL(2) V_FR(2) V_RL(2) V_RR(2)];
V_ty = [-V_FL(1) -V_FR(1) -V_RL(1) -V_RR(1)];
